simulink model "ProposedProblem1"  (R2013a)
settings: Solver=ode45  StartTime=0.0  StopTime=500  RelTol=1e-3
undefined symbols (not defined in the file): des, gcbh
settings Model: Creator=gabig  LastModifiedBy=gabig

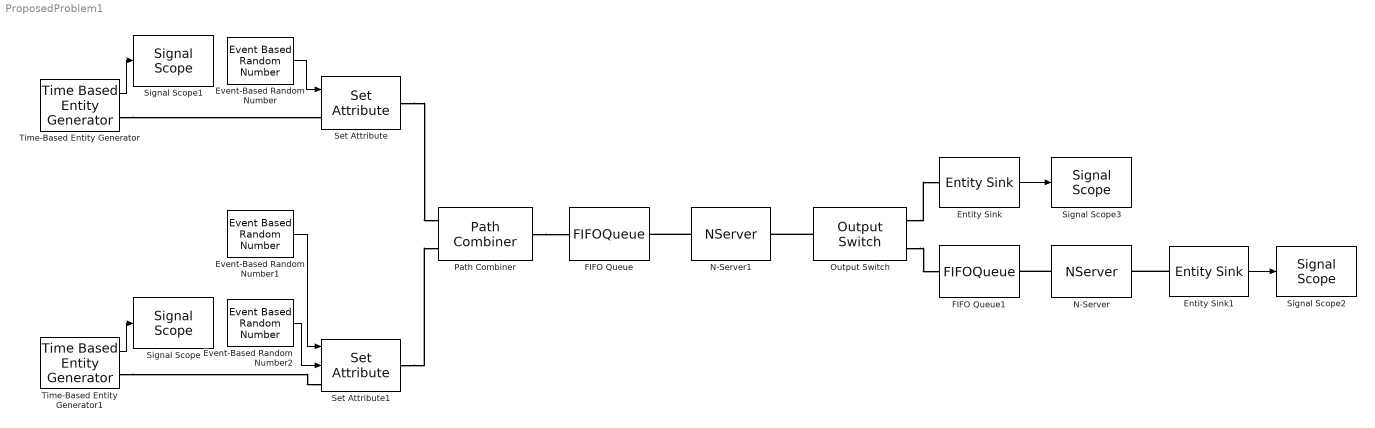
== system ProposedProblem1 ==
  Entity Sink : EntitySink  StatNumberArrived=on
  Entity Sink1 : EntitySink  StatNumberArrived=on
  Event-Based Random Number : EventBasedRandomNumber  Distribution=Uniform  minUnif=14  maxUnif=22  Seed=12322
  Event-Based Random Number1 : EventBasedRandomNumber  Distribution=Uniform  minUnif=14  maxUnif=22  Seed=12312
  Event-Based Random Number2 : EventBasedRandomNumber  Distribution=Uniform  minUnif=8  maxUnif=12  Seed=12331
  FIFO Queue : FIFOQueue
  FIFO Queue1 : FIFOQueue
  N-Server : NServer  ServiceTimeFrom=Attribute  AttributeName=WORK2
  N-Server1 : NServer  ServiceTimeFrom=Attribute  AttributeName=WORK1
  Output Switch : OutputSwitch  NumberOutputPorts=2  SwitchingCriterion=From attribute  AttributeName=LOT
  Path Combiner : PathCombiner  NumberInputPorts=2
  Set Attribute : SetAttribute  AttributeName=WORK1|LOT  AttributeFrom=Signal port|Dialog  AttributeValue=1|1  AttributeTreatAsVector=1|1  EvaluatedAttributeValue={ [];1}
  Set Attribute1 : SetAttribute  AttributeName=WORK1|WORK2|LOT  AttributeFrom=Signal port|Signal port|Dialog  AttributeValue=1|2|2  AttributeTreatAsVector=1|1|1  EvaluatedAttributeValue={ [];[];2}
      settings: InputPortMap=u0,u1
  Signal Scope{,1..3} (4 alike) : SignalScope  LoadFcn=des.scope.CallbackSupport('seLoadFcn',gcbh)  StartFcn=des.scope.CallbackSupport('seStartFcn',gcbh)  StopFcn=des.scope.CallbackSupport('seStopFcn',gcbh)
      settings: CopyFcn=des.scope.CallbackSupport('seCopyFcn',gcbh)  DeleteFcn=des.scope.CallbackSupport('seDeleteFcn',gcbh)  PreSaveFcn=des.scope.CallbackSupport('sePreSaveFcn',gcbh)  NameChangeFcn=des.scope.CallbackSupport('seNameChangeFcn',gcbh)  OpenFcn=des.scope.CallbackSupport('seOpenFcn',gcbh)
  Time-Based Entity Generator : TimeBasedEntityGenerator  Distribution=Uniform  InitialSeed=12654  Minimum=25  Maximum=45  StatNumberDeparted=on
  Time-Based Entity Generator1 : TimeBasedEntityGenerator  Distribution=Uniform  InitialSeed=12388  Minimum=38  Maximum=52  StatNumberDeparted=on
  wires:
  Time-Based Entity Generator/1 -> Signal Scope1/1
  Time-Based Entity Generator1/1 -> Signal Scope/1
  Event-Based Random Number1/1 -> Set Attribute1/1
  Entity Sink1/1 -> Signal Scope2/1
  Entity Sink/1 -> Signal Scope3/1
  Event-Based Random Number/1 -> Set Attribute/1
  Event-Based Random Number2/1 -> Set Attribute1/2
  connections:
  Set Attribute/RConn1 -- Path Combiner/LConn1
  Time-Based Entity Generator1/RConn1 -- Set Attribute1/LConn1
  Time-Based Entity Generator/RConn1 -- Set Attribute/LConn1
  N-Server1/LConn1 -- FIFO Queue/RConn1
  Path Combiner/RConn1 -- FIFO Queue/LConn1
  Entity Sink1/LConn1 -- N-Server/RConn1
  Output Switch/LConn1 -- N-Server1/RConn1
  N-Server/LConn1 -- FIFO Queue1/RConn1
  Set Attribute1/RConn1 -- Path Combiner/LConn2
  Output Switch/RConn2 -- FIFO Queue1/LConn1
  Output Switch/RConn1 -- Entity Sink/LConn1
